simulink model "Prova_es4_sim"  (R2022b)
settings: Solver=VariableStepAuto  StartTime=0.0  StopTime=10.0  RelTol=1e-3
undefined symbols (not defined in the file or in its folder): den, denF, denH, K_xi, num, numF, numH
settings Model: Creator=marcoverri  LastModifiedBy=marcoverri

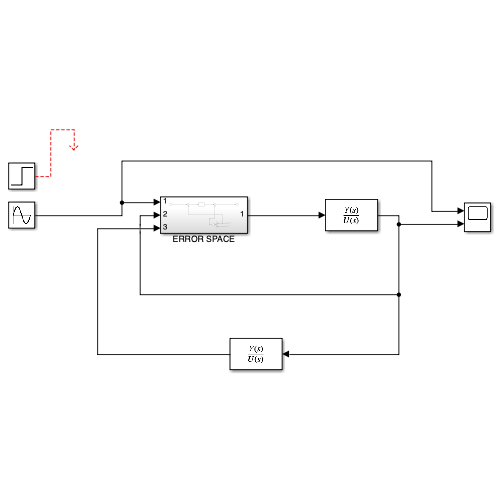
[thumbnail: Simulink's stored preview of the top-level diagram]
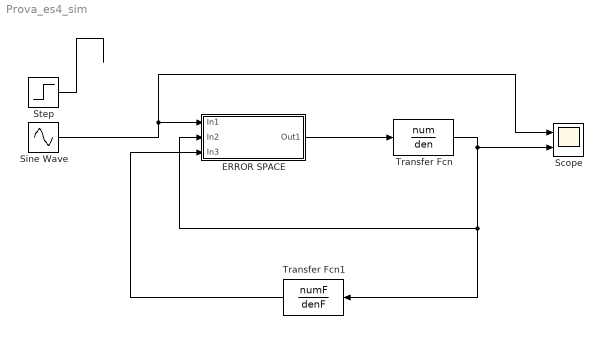
== system Prova_es4_sim ==
  ERROR SPACE : Subsystem
  Scope : Scope  NumInputPorts=2
  Sine Wave : Sin  Frequency=6  SampleTime=0
  Step : Step  SampleTime=0
  Transfer Fcn : TransferFcn  Numerator=num  Denominator=den
  Transfer Fcn1 : TransferFcn  Numerator=numF  Denominator=denF
  wires:
  ERROR SPACE/1(Out1) -> Transfer Fcn/1
  Transfer Fcn/1 -> ERROR SPACE/2(In2), Transfer Fcn1/1, Scope/2
  Transfer Fcn1/1 -> ERROR SPACE/3(In3)
  Step/1 -> ?
  Sine Wave/1 -> Scope/1, ERROR SPACE/1(In1)

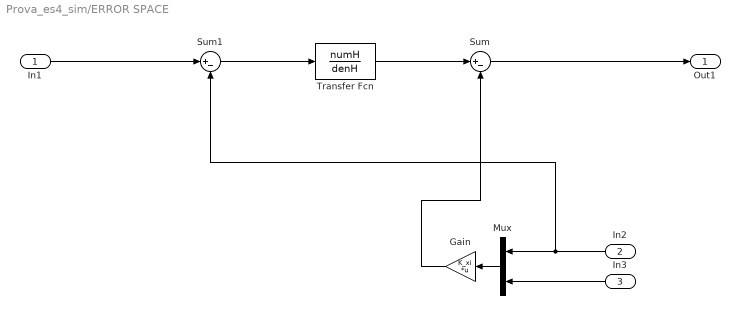
== system Prova_es4_sim/ERROR SPACE ==
  In1 : Inport
  In2 : Inport  Port=2
  In3 : Inport  Port=3
  Gain : Gain  Gain=K_xi  Multiplication=Matrix(K*u)
  Mux : Mux  Inputs=2
  Sum : Sum  Inputs=|+-
  Sum1 : Sum  Inputs=|+-
  Transfer Fcn : TransferFcn  Numerator=numH  Denominator=denH
  Out1 : Outport
  wires:
  In2/1 -> Sum1/2, Mux/1
  In3/1 -> Mux/2
  Sum1/1 -> Transfer Fcn/1
  In1/1 -> Sum1/1
  Transfer Fcn/1 -> Sum/1
  Mux/1 -> Gain/1
  Sum/1 -> Out1/1
  Gain/1 -> Sum/2
